simulink model "canPack_TBM_02"  (R2020a)
settings: Solver=VariableStepAuto  StartTime=0.0  StopTime=10.0  RelTol=1e-3
libraries: MyLibrary x1
settings Model: Creator=Administrator  LastModifiedBy=Administrator

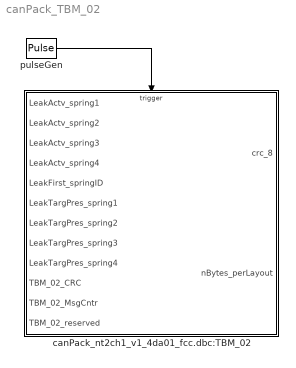
== system canPack_TBM_02 ==
  canPack_nt2ch1_v1_4da01_fcc.dbc:TBM_02 : Subsystem
  pulseGen : DiscretePulseGenerator  PulseType=Time based  Period=0.01  PulseWidth=50
  wires:
  pulseGen/1 -> canPack_nt2ch1_v1_4da01_fcc.dbc:TBM_02/Trigger

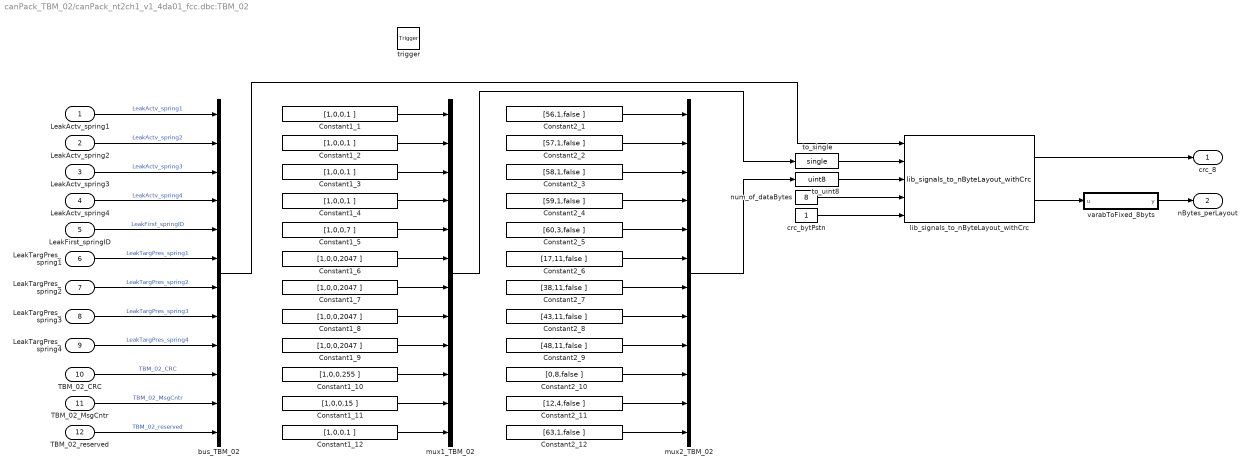
== system canPack_TBM_02/canPack_nt2ch1_v1_4da01_fcc.dbc:TBM_02 ==
  LeakActv_spring1 : Inport
  LeakActv_spring2 : Inport  Port=2
  LeakActv_spring3 : Inport  Port=3
  LeakActv_spring4 : Inport  Port=4
  LeakFirst_springID : Inport  Port=5
  LeakTargPres_spring1 : Inport  Port=6
  LeakTargPres_spring2 : Inport  Port=7
  LeakTargPres_spring3 : Inport  Port=8
  LeakTargPres_spring4 : Inport  Port=9
  TBM_02_CRC : Inport  Port=10
  TBM_02_MsgCntr : Inport  Port=11
  TBM_02_reserved : Inport  Port=12
  trigger : TriggerPort  VariantControl=Variant  PortDimensions=1
  Constant1_{1..4,12} (5 alike) : Constant  Value=[1,0,0,1 ]  SampleTime=-1
  Constant1_10 : Constant  Value=[1,0,0,255 ]  SampleTime=-1
  Constant1_11 : Constant  Value=[1,0,0,15 ]  SampleTime=-1
  Constant1_5 : Constant  Value=[1,0,0,7 ]  SampleTime=-1
  Constant1_{6..9} (4 alike) : Constant  Value=[1,0,0,2047 ]  SampleTime=-1
  Constant2_1 : Constant  Value=[56,1,false ]  SampleTime=-1
  Constant2_10 : Constant  Value=[0,8,false ]  SampleTime=-1
  Constant2_11 : Constant  Value=[12,4,false ]  SampleTime=-1
  Constant2_12 : Constant  Value=[63,1,false ]  SampleTime=-1
  Constant2_2 : Constant  Value=[57,1,false ]  SampleTime=-1
  Constant2_3 : Constant  Value=[58,1,false ]  SampleTime=-1
  Constant2_4 : Constant  Value=[59,1,false ]  SampleTime=-1
  Constant2_5 : Constant  Value=[60,3,false ]  SampleTime=-1
  Constant2_6 : Constant  Value=[17,11,false ]  SampleTime=-1
  Constant2_7 : Constant  Value=[38,11,false ]  SampleTime=-1
  Constant2_8 : Constant  Value=[43,11,false ]  SampleTime=-1
  Constant2_9 : Constant  Value=[48,11,false ]  SampleTime=-1
  bus_TBM_02 : BusCreator  Inputs=12
  crc_bytPstn : Constant  OutDataTypeStr=uint8  SampleTime=-1
  lib_signals_to_nByteLayout_withCrc : MyLibrary/lib_signals_to_nByteLayout_withCrc  SystemSampleTime=-1  Latency=0  AutoFrameSizeCalculation=off
  mux1_TBM_02 : Mux  Inputs=12
  mux2_TBM_02 : Mux  Inputs=12
  num_of_dataBytes : Constant  Value=8  OutDataTypeStr=uint8  SampleTime=-1
  to_single : DataTypeConversion  OutDataTypeStr=single
  to_uint8 : DataTypeConversion  OutDataTypeStr=uint8
  varabToFixed_8byts : MATLAB Function  TreatAsAtomicUnit=on
  crc_8 : Outport
  nBytes_perLayout : Outport  Port=2
  wires:
  LeakActv_spring1/1 -> bus_TBM_02/1  "LeakActv_spring1"
  LeakActv_spring2/1 -> bus_TBM_02/2  "LeakActv_spring2"
  LeakActv_spring3/1 -> bus_TBM_02/3  "LeakActv_spring3"
  LeakActv_spring4/1 -> bus_TBM_02/4  "LeakActv_spring4"
  LeakFirst_springID/1 -> bus_TBM_02/5  "LeakFirst_springID"
  LeakTargPres_spring1/1 -> bus_TBM_02/6  "LeakTargPres_spring1"
  LeakTargPres_spring2/1 -> bus_TBM_02/7  "LeakTargPres_spring2"
  LeakTargPres_spring3/1 -> bus_TBM_02/8  "LeakTargPres_spring3"
  LeakTargPres_spring4/1 -> bus_TBM_02/9  "LeakTargPres_spring4"
  TBM_02_CRC/1 -> bus_TBM_02/10  "TBM_02_CRC"
  TBM_02_MsgCntr/1 -> bus_TBM_02/11  "TBM_02_MsgCntr"
  TBM_02_reserved/1 -> bus_TBM_02/12  "TBM_02_reserved"
  Constant1_1/1 -> mux1_TBM_02/1
  Constant2_1/1 -> mux2_TBM_02/1
  Constant1_2/1 -> mux1_TBM_02/2
  Constant2_2/1 -> mux2_TBM_02/2
  Constant1_3/1 -> mux1_TBM_02/3
  Constant2_3/1 -> mux2_TBM_02/3
  Constant1_4/1 -> mux1_TBM_02/4
  Constant2_4/1 -> mux2_TBM_02/4
  Constant1_5/1 -> mux1_TBM_02/5
  Constant2_5/1 -> mux2_TBM_02/5
  Constant1_6/1 -> mux1_TBM_02/6
  Constant2_6/1 -> mux2_TBM_02/6
  Constant1_7/1 -> mux1_TBM_02/7
  Constant2_7/1 -> mux2_TBM_02/7
  Constant1_8/1 -> mux1_TBM_02/8
  Constant2_8/1 -> mux2_TBM_02/8
  Constant1_9/1 -> mux1_TBM_02/9
  Constant2_9/1 -> mux2_TBM_02/9
  Constant1_10/1 -> mux1_TBM_02/10
  Constant2_10/1 -> mux2_TBM_02/10
  Constant1_11/1 -> mux1_TBM_02/11
  Constant2_11/1 -> mux2_TBM_02/11
  Constant1_12/1 -> mux1_TBM_02/12
  Constant2_12/1 -> mux2_TBM_02/12
  bus_TBM_02/1 -> lib_signals_to_nByteLayout_withCrc/1
  mux1_TBM_02/1 -> to_single/1
  to_single/1 -> lib_signals_to_nByteLayout_withCrc/2
  mux2_TBM_02/1 -> to_uint8/1
  to_uint8/1 -> lib_signals_to_nByteLayout_withCrc/3
  lib_signals_to_nByteLayout_withCrc/1 -> crc_8/1
  num_of_dataBytes/1 -> lib_signals_to_nByteLayout_withCrc/4
  lib_signals_to_nByteLayout_withCrc/2 -> varabToFixed_8byts/1(u)
  varabToFixed_8byts/1(y) -> nBytes_perLayout/1
  crc_bytPstn/1 -> lib_signals_to_nByteLayout_withCrc/5

== matlab function canPack_TBM_02/canPack_nt2ch1_v1_4da01_fcc.dbc:TBM_02/varabToFixed_8byts ==
  data: u input uint8 size=8; y output uint8
function y = fcn(u)

fixed_size = 8;
y = uint8(zeros(fixed_size,1));

for i=1:fixed_size
    y(i) = u(i);
end
